simulink model "VATsimLev"  (R2017a)
settings: Solver=ode23t  StartTime=0.0  StopTime=25  FixedStep=0.001  MaxStep=0.0001  RelTol=1e-3
undefined symbols (not defined in the file): sigbuilder_block
libraries: fl_lib x8, nesl_utility x7, elec_lib x4
settings Model: Creator=usuario  LastModifiedBy=usuario
settings DebuggingCC: SFNoUnconditionalDefaultTransitionDiag=warning

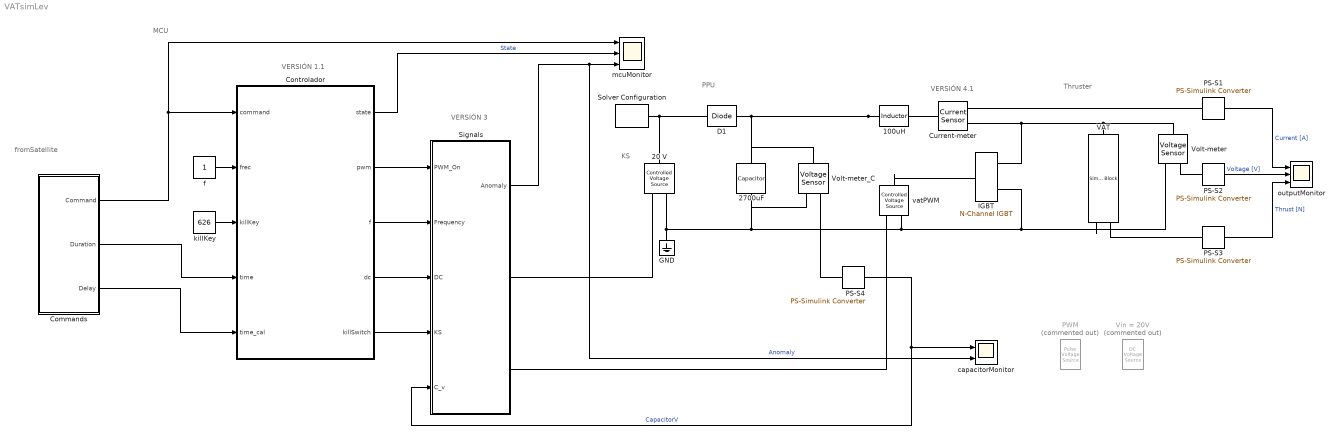
== system VATsimLev ==
  note: Thruster
  note: KS
  note: fromSatellite
  note: PPU
  note: MCU
  note: VERSIÓN 4.1
  note: VERSIÓN 1.1
  note: VERSIÓN 3
  100uH : fl_lib/Electrical/Electrical Elements/Inductor  l=100 uH  r=0.0024 Ohm  g=1e-9 1/Ohm  i_specify=off  i_priority=None  i=0 A  i_nominal_specify=off  i_nominal_unit=A  i_nominal_value=1  v_specify=off  v_priority=None  v=0 V  v_nominal_specify=off  v_nominal_unit=V  v_nominal_value=1  i_L_specify=on  i_L_priority=High  i_L=0 A  i_L_nominal_specify=off  i_L_nominal_unit=A  i_L_nominal_value=1
  20 V : fl_lib/Electrical/Electrical Sources/Controlled Voltage Source
  2700uF : fl_lib/Electrical/Electrical Elements/Capacitor  c=2700 uF  r=1e-6 Ohm  g=0 1/Ohm  i_specify=off  i_priority=None  i=0 A  i_nominal_specify=off  i_nominal_unit=A  i_nominal_value=1  v_specify=off  v_priority=None  v=0 V  v_nominal_specify=off  v_nominal_unit=V  v_nominal_value=1  vc_specify=on  vc_priority=High  vc=11.3 V  vc_nominal_specify=off  vc_nominal_unit=V  vc_nominal_value=1
  Commands : Subsystem  Tag=STV Subsys  LoadFcn=sigbuilder_block('load');  StartFcn=sigbuilder_block('start');  StopFcn=sigbuilder_block('stop');  ClipboardFcn=sigbuilder_block('clipboard');  mask(Sigbuilder block){tuvar=[0:10]}
      mask help: Simulink:masks:SigbuilderBlock_MD
      mask init:
      | if ~strcmp(get_param(bdroot(gcbh),'SimulationStatus'),'stopped') tuvar = sigbuilder_block('maskInit'); end
      settings: CopyFcn=sigbuilder_block('copy');  DeleteFcn=sigbuilder_block('delete');  ModelCloseFcn=sigbuilder_block('modelClose');  PreSaveFcn=sigbuilder_block('preSave');  PauseFcn=sigbuilder_block('pause');  ContinueFcn=sigbuilder_block('continue');  NameChangeFcn=sigbuilder_block('namechange');  OpenFcn=sigbuilder_block('open',[87 94.8 642.6 428.4 ]);  CloseFcn=sigbuilder_block('close');
      mask Display: plot(0, 0, 100, 100,[2, 2, 32, 32, 2], [68, 8, 8, 68, 68],[32, 2], [38, 38], [32, 19, 2],[53, 60, 44], [32, 17, 17, 2],[16, 16, 31, 31]);txt = getActiveGroup(gcbh);text(2, 100, txt,'verticalAlignment', 'top');
  Controlador : Stateflow chart  TreatAsAtomicUnit=on
  Current-meter : fl_lib/Electrical/Electrical Sensors/Current Sensor
  D1 : elec_lib/Semiconductor Devices/Diode  ModelType=1  Vf=0.7 V  Ron=0.3 Ohm  Goff=1e-8 S  Rz=0.3 Ohm  Vz=50 V  C_PWL=5 pF  prmExp=1  I12=[0.0137, 0.545] A  V12=[0.6, 0.7] V  I1=0.0137 A  V1=0.6 V  IS=1e-12 A  ec=1  RS=0.01 Ohm  Tmeas=25 degC  BV=inf V  C_param=1  CJ0=5 pF  VJ=1 V  Mgrad=0.5  Vvec=[0.1, 10.0, 100.0] V  Cvec=[3.5, 1.0, 0.4] pF  FC=0.5  Q_param=1  Irrm=-7.15 A  iF=4 A  didt=-750 A/us  trr=115 ns  TT=50 ns  tau=100 ns  T_param=1  IS_T2=1.25e-7 A  I1_T2=0.245 A  V1_T2=0.5 V  Tmeas2=125 degC  EG_param=1  EG=1.11 eV  XTI_param=1  XTI=3  dBVdT=0 V/K  Tdevice=25 degC  i_capacitor_specify=off  i_capacitor_priority=High  i_capacitor=0 A  i_capacitor_nominal_specify=off  i_capacitor_nominal_unit=A  i_capacitor_nominal_value=1  v_capacitor_specify=off  v_capacitor_priority=None  v_capacitor=0 V  v_capacitor_nominal_specify=off  v_capacitor_nominal_unit=V  v_capacitor_nominal_value=1  Rth=[0.0, 10.0] K/W  thermal_mass_parameterization=1  thermal_mass=[0.0, 1.0] J/K  thermal_time_constant=[0.0, 10.0] s  thermal_mass_initial_temperatures=[25.0, 25.0] degC
      settings: SourceProductName=Simscape Electronics  SourceProductBaseCode=SN
  GND : fl_lib/Electrical/Electrical Elements/Electrical Reference
  IGBT : elec_lib/Semiconductor Devices/N-Channel IGBT  model_type=1  Ices=2 mA  Vces=600 V  Vth=2 V  Vce_sat=2.6 V  Ice_sat=400 A  Vge_sat=10 V  ec=1  Tmeas=25 degC  Vge_vec=[ -2 6 7 8 10 12 15 20 ] V  Vce_vec=[ -1 0 0.5 1 1.5 2 2.5 3 3.5 4 ] V  Ic_mat=[ -1.015e-5 1.35e-8 4.7135e-4 5.092e-4 5.105e-4 5.117500000000001e-4 5.1299e-4 5.1423e-4 5.1548e-4 5.1672e-4; -9.986899999999999e-6 1.35e-8 4.7135e-4 5.092e-4 5.105e-4 5.117500000000001e-4 5.1299e-4 5.1423e-4 5.1548e-4 5.1672e-4; -9.955e-6 1.35e-8 0.0065225 3.3324 48.154 93.661 105.52 105.72 105.93 106.14; -9.955e-6 1.35e-8 0.0065235 3.5783 70.264 166.33 252.4 317.67 353.38 357.39; -9.955e-6 1.35e-8 0.006524 3.7206 89.17100000000001 228.09 371.63 511.02 642.6900000000001 764.04; -9.9549e-6 1.35e-8 0.0065242 3.7716 97.79300000000001 256.21 424.27 592.92 759.2 921.52; -9.9549e-6 1.35e-8 0.0065243 3.8067 104.52 278.11 464.6 654.37 844.5700000000001 1.0339e+3; -9.9549e-6 1.35e-8 0.0065244 3.8324 109.92 295.67 496.54 702.28 909.96 1.1183e+3 ] A  C_param=1  C_GE=23.7 nF  C_GC=2.7 nF  C_CE=0 nF  C_ies=26.4 nF  C_res=2.7 nF  C_oes=0 nF  C_GE_vec=[ 25 31 26.5 24.9 25 24.9 24.6 24.7 24.8 ] nF  C_GC_vec=[ 55 9 5.5 3.1 2.5 2.1 1.9 1.8 1.7 ] nF  C_CE_vec=[ 5 11 6.5 4.9 3.5 2.7 2.1 1.7 1.4 ] nF  C_ies_vec=[ 80 40 32 28 27.5 27 26.5 26.5 26.5 ] nF  C_res_vec=[ 55 9 5.5 3.1 2.5 2.1 1.9 1.8 1.7 ] nF  C_oes_vec=[ 60 20 12 8 6 4.8 4 3.5 3.1 ] nF  C_Vce_vec=[ 0 1 2 5 10 15 20 25 30 ] V  charge_linearity_param=1  C_OX=20 nF  V_C_OX=-5 V  TF=0 us  VAF=200 V  RC=0.001 Ohm  RE=0.001 Ohm  RG=0.001 Ohm  BF=50  T_param=1  Ices_T2=100 mA  EG=1.11 eV  Vce_sat_T2=3 V  Tmeas2=125 degC  XTI=3  BEX=-1.5  RG_alpha=0 1/K  Tdevice=25 degC  Rth=[0.0, 10.0] K/W  thermal_mass_parameterization=1  thermal_mass=[0.0, 1.0] J/K  thermal_time_constant=[0.0, 10.0] s  thermal_mass_initial_temperatures=[298.15, 298.15] K  Ic_vec1=[0.0, 10.0, 50.0, 100.0, 200.0, 400.0, 600.0] A  Vce_vec1=[0.0, 1.1, 1.3, 1.45, 1.75, 2.25, 2.7] V  Rmiller=0.1 Ohm  Goff=1e-5 1/Ohm  t_on=0.07 us  t_rise=0.7 us  t_off=0.2 us  t_fall=0.5 us  v_meas=300 V  Tj_vec1=[298.15, 398.15] K  Vce_mat1=[0.0, 1.1, 1.3, 1.45, 1.75, 2.25, 2.7; 0.0, 1.0, 1.15, 1.35, 1.7, 2.35, 3.0] V  E_turn_on_mat1=[0.0, 0.2, 1.0, 2.0, 4.0, 8.0, 15.0; 0.0, 0.3, 1.3, 2.5, 5.0, 11.0, 18.0] * 1e-3 J  E_turn_off_mat1=[0.0, 0.3, 1.5, 3.0, 6.0, 15.0, 25.0; 0.0, 0.7, 3.3, 6.5, 13.0, 25.0, 35.0] * 1e-3 J
      settings: SourceProductName=Simscape Electronics  SourceProductBaseCode=SN
  PS-S{1..4} (4 alike) : nesl_utility/PS-Simulink Converter  PhysicalDomain=network_engine_domain  SubClassName=ps_output  LeftPortType=input  RightPortType=output  PseudoPeriodic=off  Frequencies=[]  Unit=1  AffineConversion=off
  PWM : elec_lib/Additional Components/SPICE-Compatible Components/Sources/Pulse Voltage Source  Commented=on  V1=0 V  V2=5 V  TD=0.002 s  TR=1e-9 s  TF=1e-9 s  PW=820 us  PER=5 ms
      settings: SourceProductName=Simscape Electronics  SourceProductBaseCode=SN
  Signals : Subsystem
  Solver Configuration : nesl_utility/Solver Configuration  PhysicalDomain=network_engine_domain  SubClassName=solver  LeftPortType=input  RightPortType=generic  Accelerate=off  Tones=[]  Harmonics=[]  SimulateNoise=off  Profile=off  UseLocalSampling=off  EnableSwitchedLinearOptims=on  FrequencyDomain=off  UseCCode=off  RelTol=0.001  AbsTol=1e-06  MinStep=1e-09  ToWorkspace=off  RevertToSquareIcSolve=off  NumHomotopyIterations=100  PhasorMode=off  PhasorModeNumHarmonics=1  OverrideAbsTol=off  DoDC=off  ResidualTolerance=1e-09  UseLocalSolver=off  LocalSolverChoice=NE_BACKWARD_EULER_ADVANCER  LocalSolverSampleTime=0.001  DoFixedCost=off  MaxNonlinIter=3  MaxModeIter=2  LinearAlgebra=Sparse  DelaysMemoryBudget=1024  AutomaticFiltering=on  FilteringTimeConstant=0.001
  "VAT  " : SimscapeComponentBlock  SourceFile=VATswitch3  ComponentPath=VATswitch3  ComponentVariants=VATswitch3  ComponentVariantNames=VATswitch3  ClassName=VATswitch3  SchemaVersion=1  R_closed=0.01 Ohm  R_off=200 kOhm  Vd=20 V  T_closed=200 V  T_open=0 A  Thrust=24.15 mN  InitMode=switching.open  i_specify=off  i_priority=None  i=0 A  i_nominal_specify=off  i_nominal_unit=A  i_nominal_value=1  v_specify=off  v_priority=None  v=0 V  v_nominal_specify=off  v_nominal_unit=V  v_nominal_value=1
      settings: CopyFcn=simscape.engine.sli.internal.componentblockcallback(gcbh,'COPY')  PreCopyFcn=simscape.engine.sli.internal.componentblockcallback(gcbh,'PRECOPY')  PreDeleteFcn=simscape.engine.sli.internal.componentblockcallback(gcbh,'PREDELETE')
      mask Type: VAT Head
      mask Display: color('red');plot([0 1 1 0 0],[0 0 1 1 0]);plot([0.7,1],[1,0.7]);plot(-2,-1.75);plot(3, 1);disp('\n.ssc\nUnresolved')
  Vin = 20V : elec_lib/Additional Components/SPICE-Compatible Components/Sources/DC Voltage Source  Commented=on  DC=20 V
      settings: SourceProductName=Simscape Electronics  SourceProductBaseCode=SN
  Volt-meter : fl_lib/Electrical/Electrical Sensors/Voltage Sensor
  Volt-meter_C : fl_lib/Electrical/Electrical Sensors/Voltage Sensor
  capacitorMonitor : Scope  NumInputPorts=2
  f : Constant
  killKey : Constant  Value=626
  mcuMonitor : Scope  NumInputPorts=3
  outputMonitor : Scope  NumInputPorts=3
  vatPWM : fl_lib/Electrical/Electrical Sources/Controlled Voltage Source
  wires:
  killKey/1 -> Controlador/3(killKey)
  Commands/2(Duration) -> Controlador/4(time)
  Commands/3(Delay) -> Controlador/5(time_cal)
  PS-S3/1 -> outputMonitor/3  "Thrust [N]"
  PS-S1/1 -> outputMonitor/1  "Current [A]"
  PS-S2/1 -> outputMonitor/2  "Voltage [V]"
  Controlador/1(state) -> mcuMonitor/2  "State"
  Controlador/2(pwm) -> Signals/1(PWM_On)
  Controlador/5(killSwitch) -> Signals/4(KS)
  Controlador/3(f) -> Signals/2(Frequency)
  PS-S4/1 -> capacitorMonitor/1, Signals/5(C_v)  "CapacitorV"
  Signals/1(Anomaly) -> mcuMonitor/3, capacitorMonitor/2  "Anomaly"
  Controlador/4(dc) -> Signals/3(DC)
  Commands/1(Command) -> mcuMonitor/1, Controlador/1(command)
  f/1 -> Controlador/2(frec)
  connections:
  IGBT/RConn2 -- vatPWM/RConn2 -- Volt-meter_C/RConn2 -- 2700uF/RConn1 -- 20 V/RConn2 -- GND/LConn1 -- Volt-meter/RConn2 -- "VAT  "/RConn2
  100uH/LConn1 -- Volt-meter_C/LConn1 -- 2700uF/LConn1 -- D1/RConn1
  IGBT/RConn1 -- Volt-meter/LConn1 -- "VAT  "/LConn1 -- Current-meter/RConn2
  Solver Configuration/RConn1 -- 20 V/LConn1 -- D1/LConn1
  "VAT  "/RConn1 -- PS-S3/LConn1
  PS-S1/LConn1 -- Current-meter/RConn1
  Current-meter/LConn1 -- 100uH/RConn1
  Volt-meter/RConn1 -- PS-S2/LConn1
  vatPWM/LConn1 -- IGBT/LConn1
  Signals/RConn1 -- 20 V/RConn1
  vatPWM/RConn1 -- Signals/RConn2
  Volt-meter_C/RConn1 -- PS-S4/LConn1

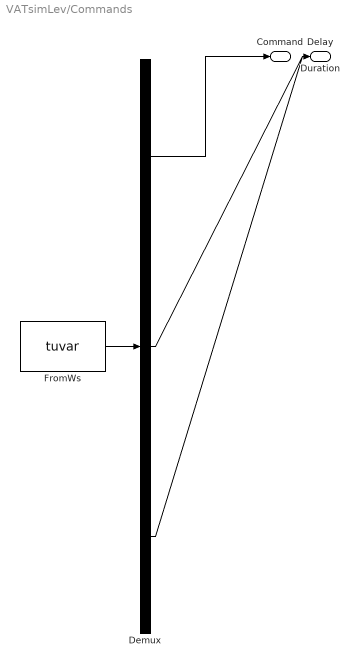
== system VATsimLev/Commands ==
  Demux : Demux  Tag=STV Demux  Outputs=3
  FromWs : FromWorkspace  Tag=STV FromWs  VariableName=tuvar  SampleTime=0
      SigBuilderData=|
      | common.afterFinalStr = 'Extrapolate'
      | common.sampleTime = 0
      | dataSet.timeRange = [0 25]
      | dataSet.name = 'Group 1'
      | sbobj.Groups.Name = 'Group 1'
      | sbobj.Groups.Signals(1).Name = 'Command'
      | sbobj.Groups.Signals(1).XData = [0 1 1 2 2 3 3 4 4 5 5 8 8 9 9 10 10 13 13 14 14 23 23 23.5 23.5 25]
      | sbobj.Groups.Signals(1).YData = [0 0 2 2 1 1 0 0 3 3 0 0 1 1 4 4 0 0 5 5 0 0 6 6 0 0]
      | sbobj.Groups.Signals(2).Name = 'Duration'
      | sbobj.Groups.Signals(2).XData = [0 9 9 10 10 13 13 14 14 25]
      | sbobj.Groups.Signals(2).YData = [0 0 3 3 0 0 4 4 0 0]
      | sbobj.Groups.Signals(3).Name = 'Delay'
      | sbobj.Groups.Signals(3).XData = [0 4 4 5 5 13 13 14 14 25]
      | sbobj.Groups.Signals(3).YData = [0 0 2 2 0 0 3 3 0 0]
      | sbobj.Groups.TimeRange = [0 25]
  Command : Outport  Tag=STV Outport
  Duration : Outport  Tag=STV Outport  Port=2
  Delay : Outport  Tag=STV Outport  Port=3
  wires:
  Demux/1 -> Command/1
  FromWs/1 -> Demux/1
  Demux/2 -> Duration/1
  Demux/3 -> Delay/1

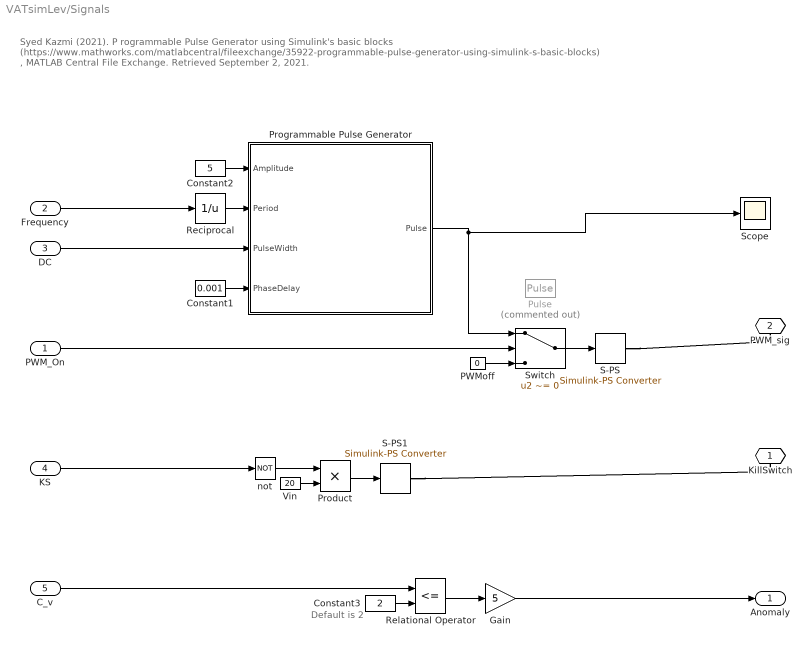
== system VATsimLev/Signals ==
  note: Default is 2
  note: Syed Kazmi (2021). P rogrammable Pulse Generator using Simulink's basic blocks
      | (https://www.mathworks.com/matlabcentral/fileexchange/35922-programmable-pulse-generator-using-simulink-s-basic-blocks)
      | , MATLAB Central File Exchange. Retrieved September 2, 2021.
  PWM_On : Inport
  Frequency : Inport  Port=2
  DC : Inport  Port=3
  KS : Inport  Port=4
  C_v : Inport  Port=5
  Constant1 : Constant  Value=0.001
  Constant2 : Constant  Value=5
  Constant3 : Constant  Value=2
  Gain : Gain  Gain=5
  PWMoff : Constant  Value=0
  Product : Product
  Programmable Pulse Generator : Subsystem
  Pulse : DiscretePulseGenerator  Commented=on  PulseType=Time based  Amplitude=5  Period=1  PulseWidth=0.082  PhaseDelay=0.001
  Reciprocal : Math  Operator=reciprocal  SaturateOnIntegerOverflow=on
  Relational Operator : RelationalOperator  Operator=<=  OutDataTypeStr=boolean  RndMeth=Simplest
  S-PS : nesl_utility/Simulink-PS Converter  PhysicalDomain=network_engine_domain  SubClassName=ps_input  LeftPortType=input  RightPortType=output  PseudoPeriodic=off  Frequencies=[]  NoiseDistribution=none  NoiseParameters=[]  Unit=1  AffineConversion=off  FilteringAndDerivatives=provide  SimscapeFilterOrder=1  InputFilterTimeConstant=0.001  UdotUserProvided=0
  S-PS1 : nesl_utility/Simulink-PS Converter  PhysicalDomain=network_engine_domain  SubClassName=ps_input  LeftPortType=input  RightPortType=output  PseudoPeriodic=off  Frequencies=[]  NoiseDistribution=none  NoiseParameters=[]  Unit=1  AffineConversion=off  FilteringAndDerivatives=zero  SimscapeFilterOrder=1  InputFilterTimeConstant=0.001  UdotUserProvided=0
  Scope : Scope
  Switch : Switch  Criteria=u2 ~= 0
  Vin : Constant  Value=20
  not : Logic  Operator=NOT  IconShape=distinctive  AllPortsSameDT=off  OutDataTypeStr=boolean
  KillSwitch : PMIOPort  Port=1  Side=Right
  PWM_sig : PMIOPort  Port=2  Side=Right
  Anomaly : Outport
  wires:
  KS/1 -> not/1
  Vin/1 -> Product/2
  PWMoff/1 -> Switch/3
  Product/1 -> S-PS1/1
  not/1 -> Product/1
  Switch/1 -> S-PS/1
  PWM_On/1 -> Switch/2
  Constant2/1 -> Programmable Pulse Generator/1(Amplitude)
  DC/1 -> Programmable Pulse Generator/3(PulseWidth)
  Constant1/1 -> Programmable Pulse Generator/4(PhaseDelay)
  Reciprocal/1 -> Programmable Pulse Generator/2(Period)
  Frequency/1 -> Reciprocal/1
  Programmable Pulse Generator/1(Pulse) -> Scope/1, Switch/1
  C_v/1 -> Relational Operator/1
  Constant3/1 -> Relational Operator/2
  Relational Operator/1 -> Gain/1
  Gain/1 -> Anomaly/1
  connections:
  S-PS/RConn1 -- PWM_sig/RConn1
  S-PS1/RConn1 -- KillSwitch/RConn1

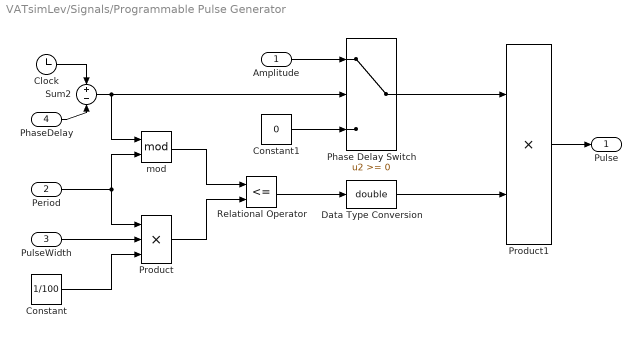
== system VATsimLev/Signals/Programmable Pulse Generator ==
  Amplitude : Inport
  Period : Inport  Port=2
  PulseWidth : Inport  Port=3
  PhaseDelay : Inport  Port=4
  Clock : Clock
  Constant : Constant  Value=1/100
  Constant1 : Constant  Value=0
  Data Type Conversion : DataTypeConversion  OutDataTypeStr=double
  Phase Delay Switch : Switch
  Product : Product  Inputs=3  RndMeth=Zero
  Product1 : Product  RndMeth=Zero
  Relational Operator : RelationalOperator  Operator=<=  RndMeth=Nearest
  Sum2 : Sum  Inputs=+-
  mod : Math  Operator=mod  SaturateOnIntegerOverflow=on
  Pulse : Outport
  wires:
  Product/1 -> Relational Operator/2
  Product1/1 -> Pulse/1
  Data Type Conversion/1 -> Product1/2
  Relational Operator/1 -> Data Type Conversion/1
  Constant/1 -> Product/3
  mod/1 -> Relational Operator/1
  Period/1 -> Product/1, mod/2
  Clock/1 -> Sum2/1
  PhaseDelay/1 -> Sum2/2
  Sum2/1 -> mod/1, Phase Delay Switch/2
  Amplitude/1 -> Phase Delay Switch/1
  Constant1/1 -> Phase Delay Switch/3
  Phase Delay Switch/1 -> Product1/1
  PulseWidth/1 -> Product/2

== stateflow chart VATsimLev/Controlador ==
  state On
    state On
      entry:
      f=frec;
      dc=0.082/(1/f);
      pwm=1;
      state=aux;
    state OnTimed
      entry:
      f=frec;
      dc=0.082/(1/f);
      pwm=1;
      state=aux;
      d=time;
      on after(d,sec):
      offFlag=1;
    (default) -> (junction 28)
    (junction 28) -> On.On [order 1] : [aux==2]
    (junction 28) -> OnTimed [order 2] : [aux==4]
  note: off				1
      | on				2
      | onCal			3
      | timedOn		4
      | timedOnCal 	5
      | kill 				6
      | setKey 		7
      | telemetry 		8
      | VATinit/null 	0
  state Scheduled
    state auxTimedCal
    state OnTimedCal
      entry:
      state=aux;
      f=frec;
      dc=0.082/(1/f);
      pwm=1;
      offFlag=0;
      on after(d,sec):
      offFlag=1;
    state OnCal
      entry:
      state=aux;
      on after(cal,sec):
      f=frec;
      dc=0.082/(1/f);
      pwm=1;
      state=aux;
    (default) -> (junction 54) : {cal=time_cal}
    (junction 54) -> auxTimedCal [order 2] : [aux == 5]{state=5; d=time}
    (junction 54) -> OnCal [order 1] : [aux==3]
    auxTimedCal -> OnTimedCal : after(cal,sec)
  state VATinit
    entry:
    key=626;
    p=0;
    state=0;
    aux=0;
    killSwitch=0;
    dc=0.1;
    f=1;
    during:
    p=1;
  state Off
    entry:
    f=1;
    dc=0.1;
    pwm=0;
    state=1;
    offFlag=0;
    aux=0;
    cal=0;
    d=0;
  state Dead
    entry:
    killSwitch = 1;
    p=0;
    f=1;
    dc=0.1;
    pwm=0;
    state=6;
    offFlag=0;
    cal=0;
    d=0;
  On -> Dead [order 2] : [command == 6 && killKey == key]
  Off -> On [order 1] : [command == 2 || command == 4]{aux=command}
  On -> Off [order 1] : [offFlag == 1 || command == 1]
  Off -> Scheduled [order 2] : [command == 3||command == 5]{aux = command}
  VATinit -> Off : [p~=0]
  (default) -> VATinit
  Scheduled -> Off [order 1] : [command == 1 || offFlag == 1]
  Off -> Dead [order 3] : [command == 6 && killKey == key]
  Scheduled -> Dead [order 2] : [command == 6 && killKey == key]
  Dead -> Dead : [command ~=0]{p=1}
  data: command input; frec input; state output; pwm output; f output; dc output; offFlag local; p local; aux local; key local; killKey input; killSwitch output; time input; d local; time_cal input; cal local
